simulink model "Slip_Ratio"  (R2020a)
settings: Solver=VariableStepAuto  StartTime=0.0  StopTime=10.0  RelTol=1e-3
settings Model: Creator=yafta  LastModifiedBy=yafta

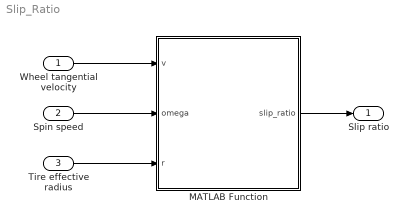
== system Slip_Ratio ==
  Wheel tangential velocity : Inport
  Spin speed : Inport  Port=2
  Tire effective radius : Inport  Port=3
  MATLAB Function : MATLAB Function  TreatAsAtomicUnit=on
  Slip ratio : Outport
  wires:
  Wheel tangential velocity/1 -> MATLAB Function/1(v)
  Spin speed/1 -> MATLAB Function/2(omega)
  Tire effective radius/1 -> MATLAB Function/3(r)
  MATLAB Function/1(slip_ratio) -> Slip ratio/1

== matlab function Slip_Ratio/MATLAB Function ==
  data: v input; slip_ratio output; omega input; r input
function slip_ratio = slip_ratio(v, omega, r)

if (omega == 0)
    slip_ratio = 0;
elseif (v == 0)
    slip_ratio = 1;
else
    slip_ratio = (omega*r-v)/v;
end
end
